simulink model "xPC_parker"  (Simulink 8.5)
settings: Solver=FixedStepDiscrete  StartTime=0.0  StopTime=inf  FixedStep=dts  RelTol=1e-3
InitFcn:
  | PARKER_DEPENDENCY
  | Parker_Multi_Axis_Init
  | Parker_ATI_Init
  | Parker_Home_Init
  | Parker_Davinci_Init
  | Parker_UDP_Init
  | Parker_LinIntPathPlan_Init
  | Parker_ScopeFormat_Init
  | Parker_magnetic_init
undefined symbols (not defined in the file): A, accel_filter_coeffs, ATI_torque_Nmm, B, counter_offset, DavinciFilterDen, DavinciFilterNum, DesiredPath, dt, dt_ENC, dt_trakstar, dts, dtudp, ENC_obs_filter_coeffs, encoder_counts, F, f_mag_desired_shape, filter_coeffs_bias, force_bias, forceDeadZone, FT_unbias_time, grav_vector, Home_in_TKbase, HOMING_dx, HOMING_num_joint, HOMING_tspan, HOMING_Vmov, inv_T, JOINT_Limits_Negative, JOINT_Limits_Postive, Kd, Ki_force, Kp, Kp_force, Kv_force, Low, N_acceleration, N_bias, N_ENC_obs_filter, N_obs_velocity, N_trakstar, N_velocity, Omega7IsLeftHanded, omni_scaling, PathPlanSpeed, pitch, quadrature_mode, R_FT2robot, R_omni, R_robot2TKbase, ResRateEpsilon, ResRateVelLimits, ResRateVelRatios, SafetyMargin, screw_pitch, torque_constant, trakstar_filter_coeffs, UDP_EN_Data2CMU, UDP_EN_DynAna, UDP_EN_VFRec ... (+6)
libraries: slrtlib x25, simulink x24, dspswit3 x15, xpcobsoletelib x15, xpcrtudplib x14, powerlib_meascontrol x3, xpcmeasurementcomputinglib x3, xpcconteclib x3
(part 1 of 3)
settings Model: Creator=Roger  LastModifiedBy=arma  CovSFcnEnable=off
settings SolverCC: EnableConcurrentExecution=on
settings OptimizationCC: BlockReduction=off  OptimizeBlockIOStorage=off  BufferReuse=off  GlobalBufferReuse=off  ExpressionFolding=off  LocalBlockOutputs=off  InitFltsAndDblsToZero=on
settings DebuggingCC: SolverPrmCheckMsg=warning  MultiTaskCondExecSysMsg=warning  MultiTaskRateTransMsg=warning  FcnCallInpInsideContextMsg=EnableAllAsWarning
settings HardwareCC: ProdIntDivRoundTo=Zero  ProdEndianess=LittleEndian  ProdLongLongMode=on  ProdHWDeviceType=Generic->32-bit x86 compatible
settings SFSimCC: SimParseCustomCode=off
settings RTWCC: SystemTargetFile=slrt.tlc  TemplateMakefile=slrt_default_tmf  Description=Simulink Real-Time  RTWCompilerOptimization=on
settings SimulinkRealTimeCC: GeneratePreprocessorConditionals=Disable all  xPCisDownloadable=off  xPCisModelTimeout=off  xPCModelTimeoutSecs=15

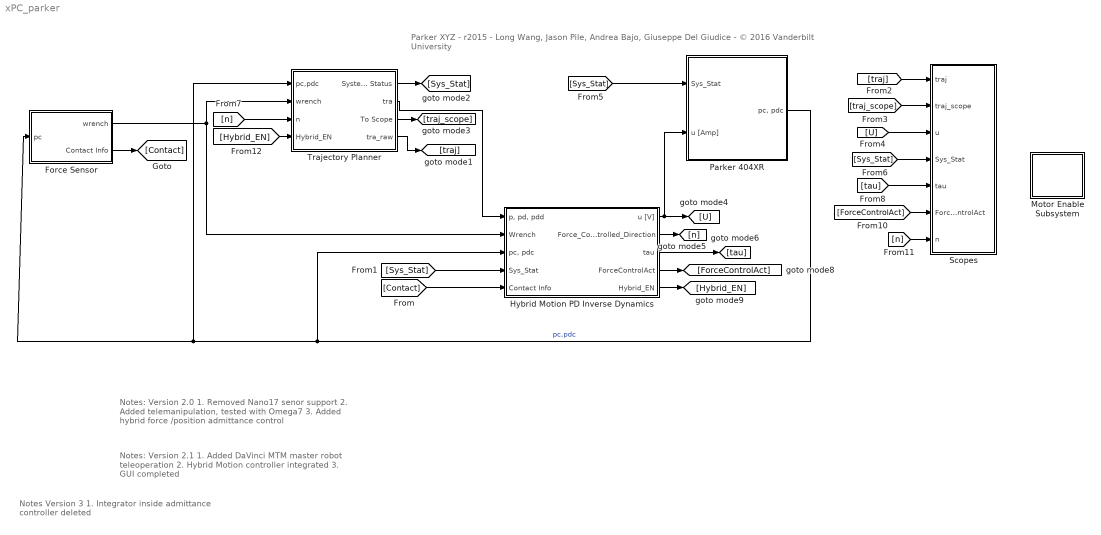
== system xPC_parker ==
  note: Notes Version 3
      | 1. Integrator inside admittance controller deleted
  note: Notes: Version 2.0
      | 1. Removed Nano17 senor support
      | 2. Added telemanipulation, tested with Omega7
      | 3. Added hybrid force /position admittance control
  note: Parker XYZ - r2015 - Long Wang, Jason Pile, Andrea Bajo, Giuseppe Del Giudice - © 2016 Vanderbilt University
  note: Notes: Version 2.1
      | 1. Added DaVinci MTM master robot teleoperation
      | 2. Hybrid Motion controller integrated
      | 3. GUI completed
  Force Sensor : Subsystem
  Hybrid Motion PD Inverse Dynamics : Subsystem  TreatAsAtomicUnit=on
  Motor Enable Subsystem : Subsystem
  Parker 404XR : Subsystem
  Scopes : Subsystem
  Trajectory Planner : Subsystem  TreatAsAtomicUnit=on
  wires:
  Hybrid Motion PD Inverse Dynamics/1(u [V]) -> [U], Parker 404XR/2(u [Amp])
  Parker 404XR/1("pc, pdc") -> Hybrid Motion PD Inverse Dynamics/3("pc, pdc"), Force Sensor/1(pc), Trajectory Planner/1(pc,pdc)  "pc,pdc"
  Trajectory Planner/2(tra) -> Hybrid Motion PD Inverse Dynamics/1("p, pd, pdd")
  Force Sensor/1(wrench) -> Hybrid Motion PD Inverse Dynamics/2(Wrench), Trajectory Planner/2(wrench)
  Trajectory Planner/1(System Status) -> [Sys_Stat]
  [Sys_Stat] -> Parker 404XR/1(Sys_Stat)
  [Sys_Stat] -> Hybrid Motion PD Inverse Dynamics/4(Sys_Stat)
  [traj] -> Scopes/1(traj)
  Trajectory Planner/3(To Scope) -> [traj_scope]
  [traj_scope] -> Scopes/2(traj_scope)
  [U] -> Scopes/3(u)
  [Sys_Stat] -> Scopes/4(Sys_Stat)
  Hybrid Motion PD Inverse Dynamics/2(Force_Controlled_Direction) -> [n]
  [n] -> Trajectory Planner/3(n)
  Hybrid Motion PD Inverse Dynamics/3(tau) -> [tau]
  [tau] -> Scopes/5(tau)
  Hybrid Motion PD Inverse Dynamics/4(ForceControlAct) -> [ForceControlAct]
  [ForceControlAct] -> Scopes/6(ForceControlAct)
  [n] -> Scopes/7(n)
  Hybrid Motion PD Inverse Dynamics/5(Hybrid_EN) -> [Hybrid_EN]
  [Hybrid_EN] -> Trajectory Planner/4(Hybrid_EN)
  Force Sensor/2(Contact Info) -> [Contact]
  [Contact] -> Hybrid Motion PD Inverse Dynamics/5(Contact Info)
  Trajectory Planner/4(tra_raw) -> [traj]

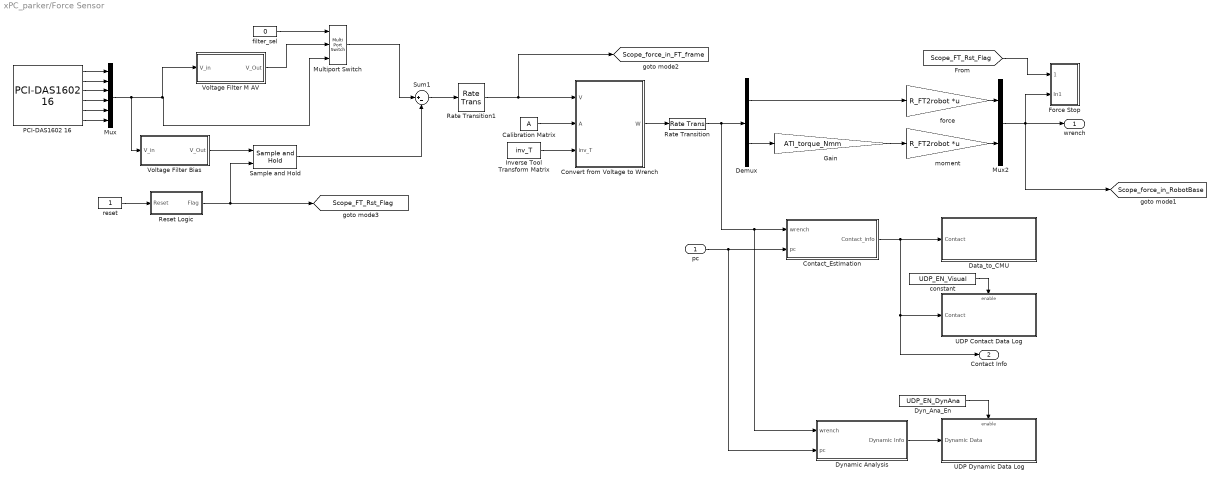
== system xPC_parker/Force Sensor ==
  pc : Inport
  Calibration Matrix : Constant  Value=A
  Contact_Estimation : Subsystem
  Convert from Voltage to Wrench : MATLAB Function  TreatAsAtomicUnit=on
  Data_to_CMU : Subsystem
  Demux : Demux  Outputs=2
  Dyn_Ana_En : Constant  Value=UDP_EN_DynAna
  Dynamic Analysis : Subsystem
  Force Stop : Subsystem
  Gain : Gain  Gain=ATI_torque_Nmm
  Inverse Tool Transform Matrix : Constant  Value=inv_T  VectorParams1D=off
  Multiport Switch : MultiPortSwitch  Inputs=2
  Mux : Mux  Inputs=6
  Mux2 : Mux  Inputs=2
  "PCI-DAS1602 16 " : xpcobsoletelib/Measurement Computing obs/A//D/PCI-DAS1602 16   channel=6  range=+-10V  mux=Differential (8 channels)  sampletime=dts  slot=-1
  Rate Transition : RateTransition  OutPortSampleTime=dt
  Rate Transition1 : RateTransition  OutPortSampleTime=dt
  Reset Logic : Subsystem
  Sample and Hold : powerlib_meascontrol/Additional Components/Sample and Hold  ic=zeros(6,1)  Ts=dts
  Sum1 : Sum  Inputs=|+-  SampleTime=dts
  UDP Contact Data Log : Subsystem
  UDP Dynamic Data Log : Subsystem
  Voltage Filter Bias : Subsystem
  Voltage Filter M AV : Subsystem
  constant : Constant  Value=UDP_EN_Visual
  filter_sel : Constant  Value=0
  force : Gain  Gain=R_FT2robot  Multiplication=Matrix(K*u)
  moment : Gain  Gain=R_FT2robot  Multiplication=Matrix(K*u)
  reset : Constant
  wrench : Outport
  Contact Info : Outport  Port=2
  tag scope: Scope_FT_Rst_Flag=global, Scope_force_in_FT_frame=global, Scope_force_in_RobotBase=global
  wires:
  "PCI-DAS1602 16 "/1 -> Mux/1
  "PCI-DAS1602 16 "/2 -> Mux/2
  "PCI-DAS1602 16 "/3 -> Mux/3
  "PCI-DAS1602 16 "/4 -> Mux/4
  "PCI-DAS1602 16 "/5 -> Mux/5
  Mux/1 -> Voltage Filter Bias/1(V_in), Voltage Filter M AV/1(V_in), Multiport Switch/3
  "PCI-DAS1602 16 "/6 -> Mux/6
  Calibration Matrix/1 -> Convert from Voltage to Wrench/2(A)
  Inverse Tool Transform Matrix/1 -> Convert from Voltage to Wrench/3(inv_T)
  Sum1/1 -> Rate Transition1/1
  Demux/1 -> force/1
  Demux/2 -> Gain/1
  force/1 -> Mux2/1
  moment/1 -> Mux2/2
  Mux2/1 -> [Scope_force_in_RobotBase], wrench/1, Force Stop/2(In1)
  Convert from Voltage to Wrench/1(W) -> Rate Transition/1
  Rate Transition/1 -> Dynamic Analysis/1(wrench), Contact_Estimation/1(wrench), Demux/1
  Multiport Switch/1 -> Sum1/1
  filter_sel/1 -> Multiport Switch/1
  Contact_Estimation/1(Contact_info) -> Contact Info/1, UDP Contact Data Log/1(Contact), Data_to_CMU/1(Contact)
  pc/1 -> Dynamic Analysis/2(pc), Contact_Estimation/2(pc)
  Voltage Filter Bias/1(V_Out) -> Sample and Hold/1
  Sample and Hold/1 -> Sum1/2
  reset/1 -> Reset Logic/1(Reset)
  Reset Logic/1(Flag) -> [Scope_FT_Rst_Flag], Sample and Hold/2
  Dynamic Analysis/1(Dynamic Info) -> UDP Dynamic Data Log/1(Dynamic Data)
  Dyn_Ana_En/1 -> UDP Dynamic Data Log/Enable
  Rate Transition1/1 -> [Scope_force_in_FT_frame], Convert from Voltage to Wrench/1(V)
  Voltage Filter M AV/1(V_Out) -> Multiport Switch/2
  constant/1 -> UDP Contact Data Log/Enable
  [Scope_FT_Rst_Flag] -> Force Stop/1(ResetFlag)
  Gain/1 -> moment/1

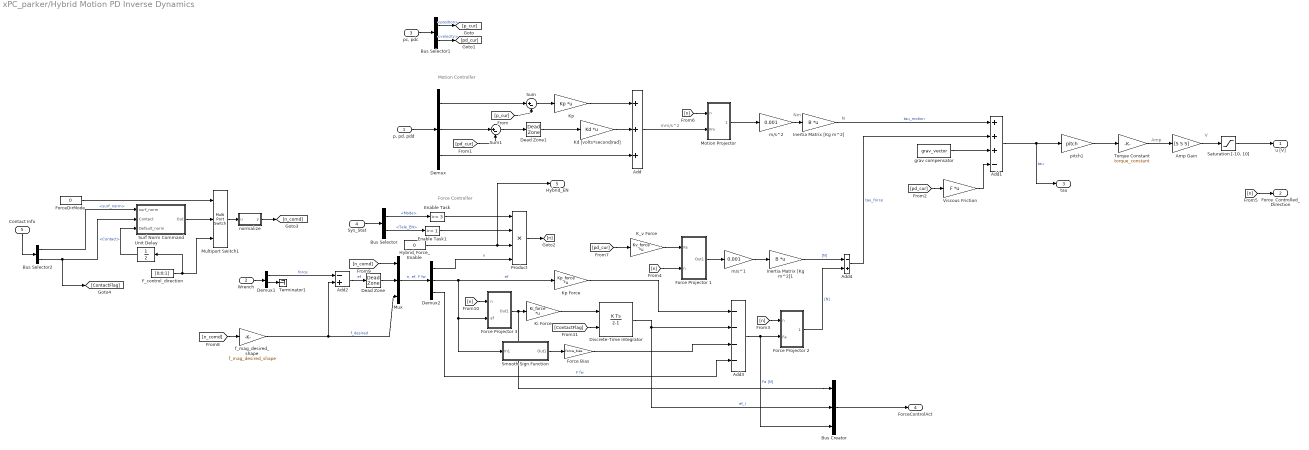
== system xPC_parker/Hybrid Motion PD Inverse Dynamics ==
  note: Force Controller
  note: Motion Controller
  note: N
  note: mm/s^2
  note: Amp
  note: V
  note: Nm
  "p, pd, pdd" : Inport
  Wrench : Inport  Port=2
  "pc, pdc" : Inport  Port=3
  Sys_Stat : Inport  Port=4
  Contact Info : Inport  Port=5
  Add : Sum  Inputs=+++
  Add1 : Sum  Inputs=+++-  SampleTime=dt
  Add2 : Sum  Inputs=-+
  Add3 : Sum  Inputs=----
  Add4 : Sum  Inputs=-+
  Amp Gain : Gain  Gain=[5 5 5]
  Bus Creator : BusCreator  Inputs=3
  Bus Selector : BusSelector  OutputSignals=Mode,Tele_EN
  Bus Selector1 : BusSelector  OutputSignals=position,velocity
  Bus Selector2 : BusSelector  OutputSignals=surf_norm,Contact
  Dead Zone : DeadZone  LowerValue=-0.02  UpperValue=0.02  SaturateOnIntegerOverflow=on
  Dead Zone1 : DeadZone  LowerValue=-2.5  UpperValue=2.5  SaturateOnIntegerOverflow=on
  Demux : Demux  Outputs=[3 3 3]
  Demux1 : Demux  Outputs=2
  Demux2 : Demux  Outputs=3
  Discrete-Time Integrator : DiscreteIntegrator  ExternalReset=falling  SampleTime=dt  UpperSaturationLimit=20  LowerSaturationLimit=-20
  Enable Task : simulink/Logic and Bit Operations/Compare To Constant  relop=>=  const=3  OutDataTypeStr=boolean
  Enable Task1 : simulink/Logic and Bit Operations/Compare To Constant  relop=>=  const=1  OutDataTypeStr=boolean
  F_control_direction : Constant  Value=[0;0;1]
  Force Bias : Gain  Gain=force_bias  SampleTime=dt
  Force Projector 1 : Subsystem  TreatAsAtomicUnit=on
  Force Projector 2 : Subsystem  TreatAsAtomicUnit=on
  Force Projector 3 : Subsystem  TreatAsAtomicUnit=on
  ForceDirMode : Constant  Value=0
  Hybrid_Force_Enable : Constant  Value=0
  Inertia Matrix [Kg m^2] : Gain  Gain=B  Multiplication=Matrix(K*u)
  Inertia Matrix [Kg m^2]1 : Gain  Gain=B  Multiplication=Matrix(K*u)
  K_v Force : Gain  Gain=Kv_force  Multiplication=Matrix(K*u)  SampleTime=dt
  Kd [volts*second/rad] : Gain  Gain=Kd  Multiplication=Matrix(K*u)
  Ki Force : Gain  Gain=Ki_force  Multiplication=Matrix(K*u)  SampleTime=dt
  Kp : Gain  Gain=Kp  Multiplication=Matrix(K*u)
  Kp Force : Gain  Gain=Kp_force  Multiplication=Matrix(K*u)  SampleTime=dt
  Motion Projector : Subsystem  TreatAsAtomicUnit=on
  Multiport Switch1 : MultiPortSwitch  Inputs=2
  Mux : Mux  Inputs=3
  Product : Product  Inputs=4  RndMeth=Zero
  "Saturation [-10, 10]" : Saturate  UpperLimit=10  LowerLimit=-10
  Smooth Sign Function : Subsystem
  Sum : Sum  Inputs=|+-
  Sum1 : Sum  Inputs=|+-
  Surf Norm Command : Subsystem
  Terminator1 : Terminator
  Torque Constant : Gain  Gain=torque_constant
  Unit Delay : UnitDelay  InitialCondition=[0;0;1]  SampleTime=-1
  Viscous Friction : Gain  Gain=F  Multiplication=Matrix(K*u)  SampleTime=dt
  f_mag_desired_shape : Gain  Gain=f_mag_desired_shape
  grav compensator : Constant  Value=grav_vector
  m/s^1 : Gain  Gain=0.001
  m/s^2 : Gain  Gain=0.001
  normalize : MATLAB Function  TreatAsAtomicUnit=on
  pitch1 : Gain  Gain=pitch
  u [V] : Outport
  Force_Controlled_Direction : Outport  Port=2
  tau : Outport  Port=3
  ForceControlAct : Outport  Port=4
  Hybrid_EN : Outport  Port=5
  wires:
  "Saturation [-10, 10]"/1 -> u [V]/1
  m/s^2/1 -> Inertia Matrix [Kg m^2]/1
  Torque Constant/1 -> Amp Gain/1
  Add1/1 -> tau/1, pitch1/1  "tau"
  pitch1/1 -> Torque Constant/1
  Amp Gain/1 -> "Saturation [-10, 10]"/1
  "p, pd, pdd"/1 -> Demux/1
  "pc, pdc"/1 -> Bus Selector1/1
  Sum/1 -> Kp/1
  Demux/1 -> Sum/1
  Demux/2 -> Sum1/1
  Bus Selector1/1 -> [p_cur]  "<position>"
  [p_cur] -> Sum/2
  [pd_cur] -> Sum1/2
  [pd_cur] -> Viscous Friction/1
  Bus Selector1/2 -> [pd_cur]  "<velocity>"
  Kp/1 -> Add/1
  Kd [volts*second/rad]/1 -> Add/2
  Demux/3 -> Add/3
  Add/1 -> Motion Projector/2(Fm)
  Motion Projector/1(Out1) -> m/s^2/1
  Ki Force/1 -> Discrete-Time Integrator/1
  Discrete-Time Integrator/1 -> Bus Creator/2, Add3/2  "ef_I"
  Demux2/2 -> Kp Force/1, Force Projector 3/2(ef), Smooth Sign Function/1(In1)  "ef"
  Kp Force/1 -> Add3/1
  Add3/1 -> Bus Creator/3, Force Projector 2/2(Fa)  "Fa [N]"
  Force Projector 1/1(Out1) -> m/s^1/1
  K_v Force/1 -> Force Projector 1/1(Fa)
  m/s^1/1 -> Inertia Matrix [Kg m^2]1/1
  Inertia Matrix [Kg m^2]1/1 -> Add4/1  "[N]"
  Force Projector 2/1(Out1) -> Add4/2  "[N]"
  Smooth Sign Function/1(Out1) -> Force Bias/1
  Force Bias/1 -> Add3/3
  Demux2/3 -> Add3/4  "F fw"
  [n] -> Force Projector 2/1(n)
  [n] -> Force Projector 1/2(n)
  [pd_cur] -> K_v Force/1
  Inertia Matrix [Kg m^2]/1 -> Add1/1  "tau_motion"
  Add4/1 -> Add1/2  "tau_force"
  grav compensator/1 -> Add1/3
  Viscous Friction/1 -> Add1/4
  f_mag_desired_shape/1 -> Add2/2, Mux/3  "f_desired"
  Add2/1 -> Dead Zone/1  "ef"
  Mux/1 -> Demux2/1  "n, ef, F fw"
  [n] -> Motion Projector/1(n)
  Wrench/1 -> Demux1/1
  Demux1/2 -> Terminator1/1
  Demux1/1 -> Add2/1  "force"
  Sys_Stat/1 -> Bus Selector/1
  Bus Selector/1 -> Enable Task/1  "<Mode>"
  Enable Task/1 -> Product/1
  Bus Selector/2 -> Enable Task1/1  "<Tele_EN>"
  [n] -> Force_Controlled_Direction/1
  Product/1 -> [n]
  Enable Task1/1 -> Product/2
  Demux2/1 -> Product/4  "n"
  Dead Zone/1 -> Mux/2
  Contact Info/1 -> Bus Selector2/1
  F_control_direction/1 -> Unit Delay/1, Multiport Switch1/3
  ForceDirMode/1 -> Multiport Switch1/1
  Multiport Switch1/1 -> normalize/1(u)
  normalize/1(y) -> [n_comd]
  [n_comd] -> f_mag_desired_shape/1
  [n_comd] -> Mux/1
  Force Projector 3/1(Out1) -> Bus Creator/1, Ki Force/1
  [n] -> Force Projector 3/1(n)
  Sum1/1 -> Dead Zone1/1
  Dead Zone1/1 -> Kd [volts*second/rad]/1
  Bus Creator/1 -> ForceControlAct/1
  Bus Selector2/2 -> Surf Norm Command/2(Contact), [ContactFlag]  "<Contact>"
  [ContactFlag] -> Discrete-Time Integrator/2
  Bus Selector2/1 -> Surf Norm Command/1(surf_norm)  "<surf_norm>"
  Surf Norm Command/1(Out) -> Multiport Switch1/2
  Unit Delay/1 -> Surf Norm Command/3(Default_norm)
  Hybrid_Force_Enable/1 -> Product/3, Hybrid_EN/1

== system xPC_parker/Motor Enable Subsystem ==
  Demux : Demux  Outputs=3
  Enable Motors : Constant  Value=ones(3,1)
  PCI-DDA08 12  to PORTA : xpcmeasurementcomputinglib/Digital Output/PCI-DDA08 12   channel=[4 5 6]  port=A  reset=[1 1 1]  initValue=[0 0 0]  chip=1  sampletime=dt  slot=-1
  wires:
  Demux/1 -> PCI-DDA08 12  to PORTA/1
  Demux/2 -> PCI-DDA08 12  to PORTA/2
  Demux/3 -> PCI-DDA08 12  to PORTA/3
  Enable Motors/1 -> Demux/1

== system xPC_parker/Parker 404XR ==
  Sys_Stat : Inport
  u [Amp] : Inport  Port=2
  Bus Creator : BusCreator  Inputs=5
  Bus Selector : BusSelector  OutputSignals=Enc_Reset
  Count to Position : Subsystem
  Magnetic Tracker 125 Hz : Subsystem  TreatAsAtomicUnit=on
      mask Display: %image(imread('trakSTAR.jpg'));
  Plant : Subsystem
  "pc, pdc" : Outport
  tag scope: Scope_p_cur=global
  wires:
  Count to Position/1(position) -> Bus Creator/1  "position"
  Plant/1(counts) -> Count to Position/1(count)
  u [Amp]/1 -> Plant/1(u)
  Bus Creator/1 -> [Scope_p_cur], "pc, pdc"/1
  Count to Position/2(velocity) -> Bus Creator/2  "velocity"
  Plant/2(LimitSW) -> Bus Creator/4  "LimitSW"
  Sys_Stat/1 -> Bus Selector/1
  Bus Selector/1 -> Count to Position/2(EncoderReset)  "<Enc_Reset>"
  Count to Position/3(acceleration) -> Bus Creator/3  "acceleration"
  Magnetic Tracker 125 Hz/1(TrakStar) -> Bus Creator/5

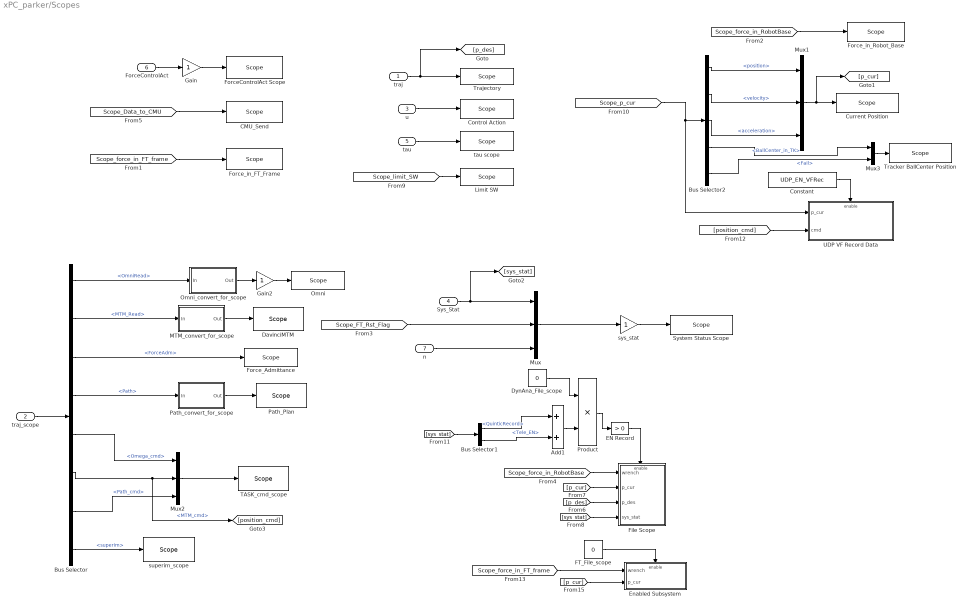
== system xPC_parker/Scopes ==
  traj : Inport
  traj_scope : Inport  Port=2
  u : Inport  Port=3
  Sys_Stat : Inport  Port=4
  tau : Inport  Port=5
  ForceControlAct : Inport  Port=6
  n : Inport  Port=7
  Add1 : Sum  SampleTime=dt
  Bus Selector : BusSelector  OutputSignals=OmniRead,MTM_Read,ForceAdm,Path,Omega_cmd,MTM_cmd,Path_cmd,superim
  Bus Selector1 : BusSelector  OutputSignals=QuinticRecord,Tele_EN
  Bus Selector2 : BusSelector  OutputSignals=position,velocity,acceleration,Tracker.BallCenter_in_TK,Tracker.Fail
  CMU_Send : slrtlib/Displays and Logging/Scope   scopeno=5  scopetype=Host  autostart=on  viewmode=Numerical  formatstr=CMU_force_scope  grid=on  ylimits=[0,0]  nosamples=Scope_Samples  noprepostsamples=0  interleave=1  triggermode=FreeRun  triggersignal=1  trigsignalfromport=off  triggerlevel=0.0  triggerslope=Either  triggerscope=1  triggersample=0  filename=data.dat  mode=Lazy  writesize=512  autorestart=off  dynamicfilemode=off  maxwritefilesize=512*1024^2
  Constant : Constant  Value=UDP_EN_VFRec
  Control Action : slrtlib/Displays and Logging/Scope   scopeno=2  scopetype=Target  autostart=on  viewmode=Numerical  formatstr=Control_Vals_format  grid=on  ylimits=[0,0]  nosamples=Scope_Samples  noprepostsamples=0  interleave=5  triggermode=FreeRun  triggersignal=1  trigsignalfromport=off  triggerlevel=0.0  triggerslope=Either  triggerscope=1  triggersample=0  filename=data.dat  mode=Lazy  writesize=512  autorestart=off  dynamicfilemode=off  maxwritefilesize=512*1024^2
  Current Position : slrtlib/Displays and Logging/Scope   scopeno=10  scopetype=Target  autostart=on  viewmode=Numerical  formatstr=Current_Position_Vals_format  grid=on  ylimits=[0,0]  nosamples=Scope_Samples  noprepostsamples=0  interleave=1  triggermode=FreeRun  triggersignal=1  trigsignalfromport=off  triggerlevel=0.0  triggerslope=Either  triggerscope=1  triggersample=0  filename=data.dat  mode=Lazy  writesize=512  autorestart=off  dynamicfilemode=off  maxwritefilesize=512*1024^2
  DavinciMTM : slrtlib/Displays and Logging/Scope   scopeno=4  scopetype=Host  autostart=on  viewmode=Numerical  formatstr=MTM_udp_scope_format  grid=on  ylimits=[0,0]  nosamples=50  noprepostsamples=0  interleave=1  triggermode=FreeRun  triggersignal=1  trigsignalfromport=off  triggerlevel=0.0  triggerslope=Either  triggerscope=1  triggersample=0  filename=data.dat  mode=Lazy  writesize=512  autorestart=off  dynamicfilemode=off  maxwritefilesize=512*1024^2
  DynAna_File_scope : Constant  Value=0
  EN Record : simulink/Logic and Bit Operations/Compare To Constant  relop=>  const=0  OutDataTypeStr=boolean
  Enabled Subsystem : Subsystem  TreatAsAtomicUnit=on
  FT_File_scope : Constant  Value=0
  File Scope : Subsystem
  ForceControlAct Scope : slrtlib/Displays and Logging/Scope   scopeno=18  scopetype=Host  autostart=on  viewmode=Numerical  formatstr=ForceControlAct_Scope  grid=on  ylimits=[0,0]  nosamples=Scope_Samples  noprepostsamples=0  interleave=1  triggermode=FreeRun  triggersignal=1  trigsignalfromport=off  triggerlevel=0.0  triggerslope=Either  triggerscope=1  triggersample=0  filename=data.dat  mode=Lazy  writesize=512  autorestart=off  dynamicfilemode=off  maxwritefilesize=512*1024^2
  Force_Admittance : slrtlib/Displays and Logging/Scope   scopeno=8  scopetype=Host  autostart=on  viewmode=Numerical  formatstr=forceAdmitFormat  grid=on  ylimits=[0,0]  nosamples=250  noprepostsamples=0  interleave=1  triggermode=FreeRun  triggersignal=1  trigsignalfromport=off  triggerlevel=0.0  triggerslope=Either  triggerscope=1  triggersample=0  filename=data.dat  mode=Lazy  writesize=512  autorestart=off  dynamicfilemode=off  maxwritefilesize=512*1024^2
  Force_in_FT_Frame : slrtlib/Displays and Logging/Scope   scopeno=6  scopetype=Host  autostart=on  viewmode=Numerical  formatstr=forceFormat  grid=on  ylimits=[0,0]  nosamples=Scope_Samples  noprepostsamples=0  interleave=1  triggermode=FreeRun  triggersignal=1  trigsignalfromport=off  triggerlevel=0.0  triggerslope=Either  triggerscope=1  triggersample=0  filename=data.dat  mode=Lazy  writesize=512  autorestart=off  dynamicfilemode=off  maxwritefilesize=512*1024^2
  Force_in_Robot_Base : slrtlib/Displays and Logging/Scope   scopeno=7  scopetype=Target  autostart=on  viewmode=Numerical  formatstr=forceFormat  grid=on  ylimits=[0,0]  nosamples=Scope_Samples  noprepostsamples=0  interleave=1  triggermode=FreeRun  triggersignal=1  trigsignalfromport=off  triggerlevel=0.0  triggerslope=Either  triggerscope=1  triggersample=0  filename=data.dat  mode=Lazy  writesize=512  autorestart=off  dynamicfilemode=off  maxwritefilesize=512*1024^2
  Gain : Gain
  Gain2 : Gain
  Limit SW : slrtlib/Displays and Logging/Scope   scopeno=9  scopetype=Host  autostart=on  viewmode=Numerical  formatstr=limitSwitchFormat  grid=on  ylimits=[0,0]  nosamples=250  noprepostsamples=0  interleave=1  triggermode=FreeRun  triggersignal=1  trigsignalfromport=off  triggerlevel=0.0  triggerslope=Either  triggerscope=1  triggersample=0  filename=data.dat  mode=Lazy  writesize=512  autorestart=off  dynamicfilemode=off  maxwritefilesize=512*1024^2
  MTM_convert_for_scope : Subsystem
  Mux : Mux  Inputs=3
  Mux1 : Mux  Inputs=3
  Mux2 : Mux  Inputs=3
  Mux3 : Mux  Inputs=2
  Omni : slrtlib/Displays and Logging/Scope   scopeno=3  scopetype=Host  autostart=on  viewmode=Numerical  formatstr=omniFormat  grid=on  ylimits=[0,0]  nosamples=50  noprepostsamples=0  interleave=1  triggermode=FreeRun  triggersignal=1  trigsignalfromport=off  triggerlevel=0.0  triggerslope=Either  triggerscope=1  triggersample=0  filename=data.dat  mode=Lazy  writesize=512  autorestart=off  dynamicfilemode=off  maxwritefilesize=512*1024^2
  Omni_convert_for_scope : Subsystem
  Path_Plan : slrtlib/Displays and Logging/Scope   scopeno=17  scopetype=Host  autostart=on  viewmode=Numerical  formatstr=Scope_format_Path  grid=on  ylimits=[0,0]  nosamples=50  noprepostsamples=0  interleave=1  triggermode=FreeRun  triggersignal=1  trigsignalfromport=off  triggerlevel=0.0  triggerslope=Either  triggerscope=1  triggersample=0  filename=data.dat  mode=Lazy  writesize=512  autorestart=off  dynamicfilemode=off  maxwritefilesize=512*1024^2
  Path_convert_for_scope : Subsystem
  Product : Product  RndMeth=Zero
  System Status Scope : slrtlib/Displays and Logging/Scope   scopeno=11  scopetype=Target  autostart=on  viewmode=Numerical  formatstr=Scope_format_sys_stat  grid=on  ylimits=[0,0]  nosamples=Scope_Samples  noprepostsamples=0  interleave=1  triggermode=FreeRun  triggersignal=1  trigsignalfromport=off  triggerlevel=0.0  triggerslope=Either  triggerscope=1  triggersample=0  filename=data.dat  mode=Lazy  writesize=512  autorestart=off  dynamicfilemode=off  maxwritefilesize=512*1024^2
  TASK_cmd_scope : slrtlib/Displays and Logging/Scope   scopeno=15  scopetype=Host  autostart=on  viewmode=Numerical  formatstr=Scope_format_TASK_cmd  grid=on  ylimits=[0,0]  nosamples=50  noprepostsamples=0  interleave=1  triggermode=FreeRun  triggersignal=1  trigsignalfromport=off  triggerlevel=0.0  triggerslope=Either  triggerscope=1  triggersample=0  filename=data.dat  mode=Lazy  writesize=512  autorestart=off  dynamicfilemode=off  maxwritefilesize=512*1024^2
  Tracker BallCenter Position : slrtlib/Displays and Logging/Scope   scopeno=21  scopetype=Host  autostart=on  viewmode=Numerical  formatstr=Scope_format_Tracker_BallCenter  grid=on  ylimits=[0,0]  nosamples=Scope_Samples  noprepostsamples=0  interleave=1  triggermode=FreeRun  triggersignal=1  trigsignalfromport=off  triggerlevel=0.0  triggerslope=Either  triggerscope=1  triggersample=0  filename=data.dat  mode=Lazy  writesize=512  autorestart=off  dynamicfilemode=off  maxwritefilesize=512*1024^2
  Trajectory : slrtlib/Displays and Logging/Scope   scopeno=1  scopetype=Target  autostart=on  viewmode=Numerical  formatstr=p_cmd_scope_format  grid=on  ylimits=[0,0]  nosamples=25  noprepostsamples=0  interleave=1  triggermode=FreeRun  triggersignal=1  trigsignalfromport=off  triggerlevel=0.0  triggerslope=Either  triggerscope=1  triggersample=0  filename=foamdata1.dat  mode=Lazy  writesize=512  autorestart=off  dynamicfilemode=off  maxwritefilesize=512*1024^2
  UDP VF Record Data : Subsystem
  superim_scope : slrtlib/Displays and Logging/Scope   scopeno=19  scopetype=Host  autostart=on  viewmode=Numerical  formatstr=Scope_format_superim  grid=on  ylimits=[0,0]  nosamples=50  noprepostsamples=0  interleave=1  triggermode=FreeRun  triggersignal=1  trigsignalfromport=off  triggerlevel=0.0  triggerslope=Either  triggerscope=1  triggersample=0  filename=data.dat  mode=Lazy  writesize=512  autorestart=off  dynamicfilemode=off  maxwritefilesize=512*1024^2
  sys_stat : Gain
  tau scope : slrtlib/Displays and Logging/Scope   scopeno=12  scopetype=Host  autostart=on  viewmode=Numerical  formatstr=Scope_format_tau  grid=on  ylimits=[0,0]  nosamples=Scope_Samples  noprepostsamples=0  interleave=1  triggermode=FreeRun  triggersignal=1  trigsignalfromport=off  triggerlevel=0.0  triggerslope=Either  triggerscope=1  triggersample=0  filename=data.dat  mode=Lazy  writesize=512  autorestart=off  dynamicfilemode=off  maxwritefilesize=512*1024^2
  wires:
  [Scope_Data_to_CMU] -> CMU_Send/1
  [Scope_force_in_FT_frame] -> Force_in_FT_Frame/1
  [Scope_force_in_RobotBase] -> Force_in_Robot_Base/1
  traj/1 -> [p_des], Trajectory/1
  Bus Selector/1 -> Omni_convert_for_scope/1(In)  "<OmniRead>"
  Bus Selector/3 -> Force_Admittance/1  "<ForceAdm>"
  u/1 -> Control Action/1
  [Scope_limit_SW] -> Limit SW/1
  traj_scope/1 -> Bus Selector/1
  Bus Selector/2 -> MTM_convert_for_scope/1(In)  "<MTM_Read>"
  MTM_convert_for_scope/1(Out) -> DavinciMTM/1
  Omni_convert_for_scope/1(Out) -> Gain2/1
  Sys_Stat/1 -> Mux/1, [sys_stat]
  Gain2/1 -> Omni/1
  tau/1 -> tau scope/1
  [Scope_FT_Rst_Flag] -> Mux/2
  Mux/1 -> sys_stat/1
  Mux1/1 -> [p_cur], Current Position/1
  Bus Selector/4 -> Path_convert_for_scope/1(In)  "<Path>"
  Path_convert_for_scope/1(Out) -> Path_Plan/1
  [Scope_force_in_RobotBase] -> File Scope/1(wrench)
  [p_cur] -> File Scope/2(p_cur)
  [p_des] -> File Scope/3(p_des)
  [sys_stat] -> File Scope/4(sys_stat)
  [sys_stat] -> Bus Selector1/1
  Bus Selector1/2 -> Add1/2  "<Tele_EN>"
  EN Record/1 -> File Scope/Enable
  [Scope_p_cur] -> UDP VF Record Data/1(p_cur), Bus Selector2/1
  Bus Selector2/1 -> Mux1/1  "<position>"
  Bus Selector2/2 -> Mux1/2  "<velocity>"
  Bus Selector2/3 -> Mux1/3  "<acceleration>"
  Bus Selector1/1 -> Add1/1  "<QuinticRecord>"
  DynAna_File_scope/1 -> Product/1
  Add1/1 -> Product/2
  Product/1 -> EN Record/1
  ForceControlAct/1 -> Gain/1
  Gain/1 -> ForceControlAct Scope/1
  Bus Selector/6 -> [position_cmd], Mux2/2  "<MTM_cmd>"
  Bus Selector/7 -> Mux2/3  "<Path_cmd>"
  Bus Selector/5 -> Mux2/1  "<Omega_cmd>"
  Mux2/1 -> TASK_cmd_scope/1
  [position_cmd] -> UDP VF Record Data/2(cmd)
  Constant/1 -> UDP VF Record Data/Enable
  Bus Selector/8 -> superim_scope/1  "<superim>"
  sys_stat/1 -> System Status Scope/1
  Bus Selector2/5 -> Mux3/2  "<Fail>"
  Bus Selector2/4 -> Mux3/1  "<BallCenter_in_TK>"
  Mux3/1 -> Tracker BallCenter Position/1
  n/1 -> Mux/3
  [Scope_force_in_FT_frame] -> Enabled Subsystem/1(wrench)
  [p_cur] -> Enabled Subsystem/2(p_cur)
  FT_File_scope/1 -> Enabled Subsystem/Enable

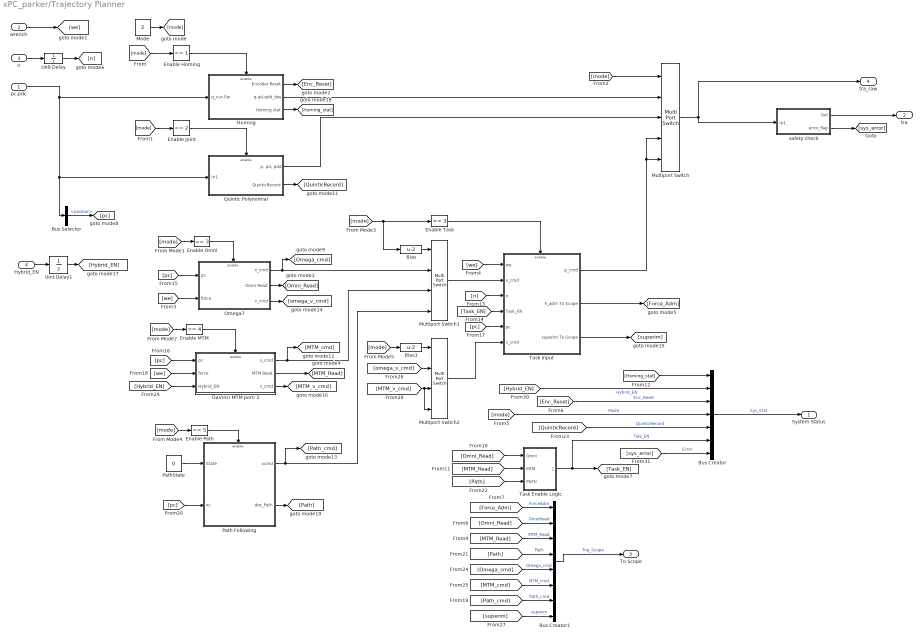
== system xPC_parker/Trajectory Planner ==
  pc,pdc : Inport
  wrench : Inport  Port=2
  n : Inport  Port=3
  Hybrid_EN : Inport  Port=4
  Bias : Bias  Bias=-2
  Bias1 : Bias  Bias=-2
  Bus Creator : BusCreator  Inputs=7
  Bus Creator1 : BusCreator  Inputs=8
  Bus Selector : BusSelector  OutputSignals=position
  DaVinci MTM port: 2 : Subsystem
  Enable Homing : simulink/Logic and Bit Operations/Compare To Constant  relop===  const=1  OutDataTypeStr=boolean
  Enable Joint : simulink/Logic and Bit Operations/Compare To Constant  relop===  const=2  OutDataTypeStr=boolean
  Enable MTM : simulink/Logic and Bit Operations/Compare To Constant  relop===  const=4  OutDataTypeStr=boolean
  Enable Omni : simulink/Logic and Bit Operations/Compare To Constant  relop===  const=3  OutDataTypeStr=boolean
  Enable Path : simulink/Logic and Bit Operations/Compare To Constant  relop===  const=5  OutDataTypeStr=boolean
  Enable Task : simulink/Logic and Bit Operations/Compare To Constant  relop=>=  const=3  OutDataTypeStr=boolean
  Homing : Subsystem
  Mode : Constant  Value=2
  Multiport Switch : MultiPortSwitch  Inputs=4
  Multiport Switch1 : MultiPortSwitch
  Multiport Switch2 : MultiPortSwitch
  Omega7 : Subsystem
  Path Following : Subsystem
  PathState : Constant  Value=0
  Quintic Polynomial : Subsystem  TreatAsAtomicUnit=on
  Task Enable Logic : Subsystem
  Task Input : Subsystem  TreatAsAtomicUnit=on
  Unit Delay : UnitDelay  InitialCondition=zeros(3,1)  SampleTime=-1
  Unit Delay1 : UnitDelay  SampleTime=-1
  safety check : Subsystem
  System Status : Outport
  tra : Outport  Port=2
  To Scope : Outport  Port=3
  tra_raw : Outport  Port=4
  wires:
  pc,pdc/1 -> Bus Selector/1, Quintic Polynomial/1(In1), Homing/1(q_cur,Sw)
  Enable Joint/1 -> Quintic Polynomial/Enable
  Homing/2(q,qd,qdd_des) -> Multiport Switch/2
  Quintic Polynomial/1("p, pd, pdd") -> Multiport Switch/3
  Enable Homing/1 -> Homing/Enable
  Mode/1 -> [mode]
  [mode] -> Enable Homing/1
  [mode] -> Enable Joint/1
  [mode] -> Multiport Switch/1
  Omega7/1(x_cmd) -> [Omega_cmd], Multiport Switch1/2
  Enable Task/1 -> Task Input/Enable
  Task Input/1(p_cmd) -> Multiport Switch/4, Multiport Switch/5
  Bus Selector/1 -> [pc]  "<position>"
  Multiport Switch1/1 -> Task Input/2(x_cmd)
  Bias/1 -> Multiport Switch1/1
  [mode] -> Enable Omni/1
  Enable Omni/1 -> Omega7/Enable
  [mode] -> Bias/1, Enable Task/1
  DaVinci MTM port: 2/1(x_cmd) -> [MTM_cmd], Multiport Switch1/3
  [mode] -> Enable MTM/1
  Enable MTM/1 -> DaVinci MTM port: 2/Enable
  wrench/1 -> [we]
  [we] -> Task Input/1(we)
  [we] -> Omega7/2(force)
  Bus Creator/1 -> System Status/1  "Sys_Stat"
  Homing/1(Encoder Reset) -> [Enc_Reset]
  [mode] -> Bus Creator/4  "Mode"
  [Enc_Reset] -> Bus Creator/3  "Enc_Reset"
  Bus Creator1/1 -> To Scope/1  "Traj_Scope"
  Omega7/2(Omni Read) -> [Omni_Read]
  DaVinci MTM port: 2/2(MTM Read) -> [MTM_Read]
  Task Input/2(F_adm To Scope) -> [Force_Adm]
  [Force_Adm] -> Bus Creator1/1  "ForceAdm"
  [Omni_Read] -> Bus Creator1/2  "OmniRead"
  [MTM_Read] -> Bus Creator1/3  "MTM_Read"
  [Omni_Read] -> Task Enable Logic/1(Omni)
  [MTM_Read] -> Task Enable Logic/2(MTM)
  Task Enable Logic/1(TeleEN) -> Bus Creator/6, [Task_EN]  "Tele_EN"
  [n] -> Task Input/3(n)
  n/1 -> Unit Delay/1
  Unit Delay/1 -> [n]
  [Task_EN] -> Task Input/4(Task_EN)
  [pc] -> Omega7/1(pc)
  [pc] -> DaVinci MTM port: 2/1(pc)
  [pc] -> Task Input/5(pc)
  [we] -> DaVinci MTM port: 2/2(force)
  PathState/1 -> Path Following/1(State)
  [pc] -> Path Following/2(xc)
  [mode] -> Enable Path/1
  Enable Path/1 -> Path Following/Enable
  Path Following/1(xcmd) -> Multiport Switch1/4, [Path_cmd]
  Path Following/2(des_Path) -> [Path]
  [Path] -> Bus Creator1/4  "Path"
  [Path] -> Task Enable Logic/3(PATH)
  Quintic Polynomial/2(QuinticRecord) -> [QuinticRecord]
  [QuinticRecord] -> Bus Creator/5  "QuinticRecord"
  [Omega_cmd] -> Bus Creator1/5  "Omega_cmd"
  [Path_cmd] -> Bus Creator1/7  "Path_cmd"
  [MTM_cmd] -> Bus Creator1/6  "MTM_cmd"
  Omega7/3(v_cmd) -> [omega_v_cmd]
  Task Input/3(superim To Scope) -> [superim]
  [superim] -> Bus Creator1/8  "superim"
  DaVinci MTM port: 2/3(v_cmd) -> [MTM_v_cmd]
  [omega_v_cmd] -> Multiport Switch2/2
  [MTM_v_cmd] -> Multiport Switch2/4, Multiport Switch2/3
  Bias1/1 -> Multiport Switch2/1
  [mode] -> Bias1/1
  Multiport Switch2/1 -> Task Input/6(v_cmd)
  Hybrid_EN/1 -> Unit Delay1/1
  [Hybrid_EN] -> DaVinci MTM port: 2/3(Hybrid_EN)
  [Hybrid_EN] -> Bus Creator/2  "Hybrid_EN"
  Unit Delay1/1 -> [Hybrid_EN]
  Homing/3(Homing stat) -> [Homing_stat]
  [Homing_stat] -> Bus Creator/1
  Multiport Switch/1 -> tra_raw/1, safety check/1(In1)
  safety check/1(Out) -> tra/1
  safety check/2(error_flag) -> [sys_error]
  [sys_error] -> Bus Creator/7  "Error"

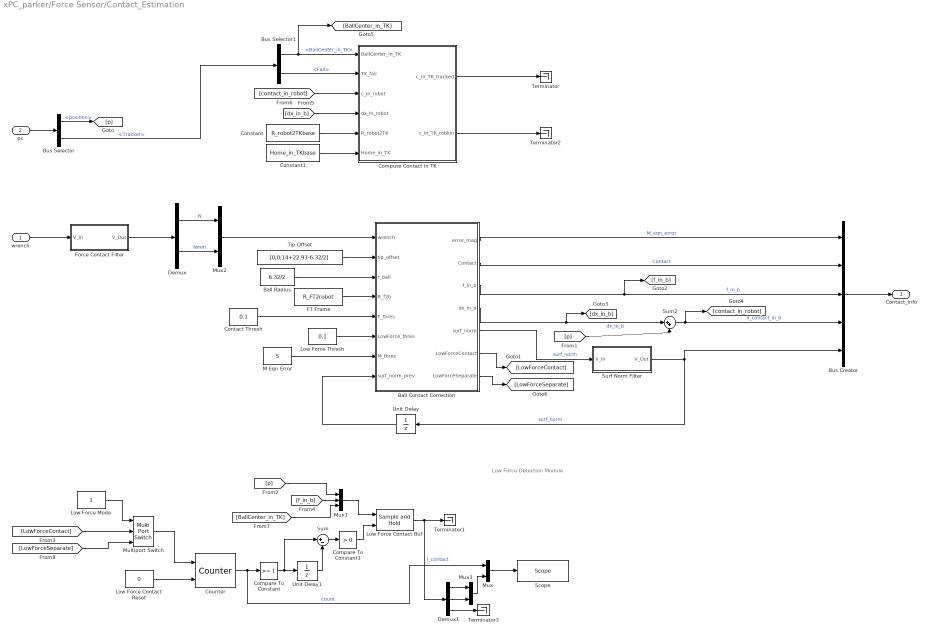
== system xPC_parker/Force Sensor/Contact_Estimation ==
  note: Low Force Detection Module
  wrench : Inport
  pc : Inport  Port=2
  Ball Contact Correction : MATLAB Function  TreatAsAtomicUnit=on
  Ball Radius : Constant  Value=6.32/2
  Bus Creator : BusCreator  Inputs=5
  Bus Selector : BusSelector  OutputSignals=position,Tracker
  Bus Selector1 : BusSelector  OutputSignals=BallCenter_in_TK,Fail
  Compare To Constant : simulink/Logic and Bit Operations/Compare To Constant  relop=>=  const=1  OutDataTypeStr=boolean
  Compare To Constant1 : simulink/Logic and Bit Operations/Compare To Constant  relop=>  const=0  OutDataTypeStr=boolean
  Compute Contact in TK : MATLAB Function  TreatAsAtomicUnit=on
  Constant : Constant  Value=R_robot2TKbase
  Constant1 : Constant  Value=Home_in_TKbase
  Contact Thresh : Constant  Value=0.1
  Counter : dspswit3/Counter  Direction=Up  CountEvent=Rising edge  CounterSize=32 bits  MaxCount=255  InitialCount=0  Output=Count  HitValue=32  ResetInput=on  SamplesPerFrame=1  Ts=1  CntDtype=double  HitDtype=Logical
  Demux : Demux  Outputs=2
  Demux1 : Demux  Outputs=[3,3,3]
  FT Frame : Constant  Value=R_FT2robot
  Force Contact Filter : Subsystem
  Low Force Contact Buf : powerlib_meascontrol/Additional Components/Sample and Hold  ic=zeros(9,1)  Ts=dt
  Low Force Contact Reset : Constant  Value=0
  Low Force Mode : Constant
  Low Force Thresh : Constant  Value=0.1
  M Eqn Error : Constant  Value=5
  Multiport Switch : MultiPortSwitch  Inputs=2
  Mux : Mux  Inputs=2
  Mux1 : Mux  Inputs=3
  Mux2 : Mux  Inputs=2
  Mux3 : Mux  Inputs=2
  "Scope " : slrtlib/Displays and Logging/Scope   scopeno=20  scopetype=Target  autostart=on  viewmode=Numerical  formatstr=Scope_format_LowForceContact  grid=on  ylimits=[0,0]  nosamples=25  noprepostsamples=0  interleave=1  triggermode=FreeRun  triggersignal=1  trigsignalfromport=off  triggerlevel=0.0  triggerslope=Either  triggerscope=1  triggersample=0  filename=data.dat  mode=Lazy  writesize=512  autorestart=off  dynamicfilemode=off  maxwritefilesize=512*1024^2
  Sum : Sum  Inputs=|+-
  Sum2 : Sum  Inputs=|++  SampleTime=dts
  Surf Norm Filter : Subsystem
  Terminator{,1..3} (4 alike) : Terminator
  Tip Offset : Constant  Value=[0;0;14+22.93-6.32/2]
  Unit Delay : UnitDelay  InitialCondition=[0;0;1]  SampleTime=-1
  Unit Delay1 : UnitDelay  SampleTime=-1
  Contact_info : Outport
  wires:
  Ball Contact Correction/2(Contact) -> Bus Creator/2  "Contact"
  FT Frame/1 -> Ball Contact Correction/4(R_f2b)
  Ball Contact Correction/1(error_mag) -> Bus Creator/1  "M_eqn_error"
  Ball Contact Correction/5(surf_norm) -> Surf Norm Filter/1(V_in)  "surf_norm"
  Ball Contact Correction/3(f_in_b) -> [f_in_b], Bus Creator/3  "f_in_b"
  Ball Radius/1 -> Ball Contact Correction/3(r_ball)
  Tip Offset/1 -> Ball Contact Correction/2(tip_offset)
  Bus Creator/1 -> Contact_info/1
  wrench/1 -> Force Contact Filter/1(V_in)
  Ball Contact Correction/4(dx_in_b) -> [dx_in_b], Sum2/1  "dx_in_b"
  Sum2/1 -> Bus Creator/4, [contact_in_robot]  "x_contact_in_b"
  Contact Thresh/1 -> Ball Contact Correction/5(F_thres)
  M Eqn Error/1 -> Ball Contact Correction/7(M_thres)
  [p] -> Sum2/2
  Force Contact Filter/1(V_Out) -> Demux/1
  Demux/2 -> Mux2/2  "Nmm"
  pc/1 -> Bus Selector/1
  Demux/1 -> Mux2/1  "N"
  Mux2/1 -> Ball Contact Correction/1(wrench)
  Bus Selector/1 -> [p]  "<position>"
  Surf Norm Filter/1(V_Out) -> Unit Delay/1, Bus Creator/5  "surf_norm"
  Unit Delay/1 -> Ball Contact Correction/8(surf_norm_prev)
  Low Force Thresh/1 -> Ball Contact Correction/6(LowForce_thres)
  Ball Contact Correction/6(LowForceContact) -> [LowForceContact]
  Low Force Contact Buf/1 -> Demux1/1, Terminator1/1  "l_contact"
  Low Force Contact Reset/1 -> Counter/2
  Mux/1 -> "Scope "/1
  Counter/1 -> Mux/1, Compare To Constant/1  "count"
  Unit Delay1/1 -> Sum/2
  Compare To Constant/1 -> Sum/1, Unit Delay1/1
  Sum/1 -> Compare To Constant1/1
  Compare To Constant1/1 -> Low Force Contact Buf/2
  [p] -> Mux1/1
  [f_in_b] -> Mux1/2
  Mux1/1 -> Low Force Contact Buf/1
  Bus Selector/2 -> Bus Selector1/1  "<Tracker>"
  Bus Selector1/1 -> [BallCenter_in_TK], Compute Contact in TK/1(BallCenter_in_TK)  "<BallCenter_in_TK>"
  Bus Selector1/2 -> Compute Contact in TK/2(TK_fail)  "<Fail>"
  [dx_in_b] -> Compute Contact in TK/4(dx_in_robot)
  Constant/1 -> Compute Contact in TK/5(R_robot2TK)
  Constant1/1 -> Compute Contact in TK/6(Home_in_TK)
  [contact_in_robot] -> Compute Contact in TK/3(c_in_robot)
  Compute Contact in TK/1(c_in_TK_tracked) -> Terminator/1
  Compute Contact in TK/2(c_in_TK_robkin) -> Terminator2/1
  [BallCenter_in_TK] -> Mux1/3
  Demux1/1 -> Mux3/1
  Demux1/2 -> Mux3/2
  Mux3/1 -> Mux/2
  Demux1/3 -> Terminator3/1
  Ball Contact Correction/7(LowForceSeparate) -> [LowForceSeparate]
  [LowForceSeparate] -> Multiport Switch/3
  [LowForceContact] -> Multiport Switch/2
  Multiport Switch/1 -> Counter/1
  Low Force Mode/1 -> Multiport Switch/1

== system xPC_parker/Force Sensor/Data_to_CMU ==
  Contact : Inport
  Bus Selector1 : BusSelector  OutputSignals=M_eqn_error,Contact,f_in_b,x_contact_in_b
  Constant : Constant  Value=UDP_EN_Data2CMU
  Mux1 : Mux  Inputs=5
  UDP : Subsystem
  tag scope: Scope_Data_to_CMU=global
  wires:
  UDP/1(delay in ms) -> Mux1/5
  Mux1/1 -> [Scope_Data_to_CMU]
  Bus Selector1/1 -> Mux1/1  "<M_eqn_error>"
  Bus Selector1/2 -> [Contact]  "<Contact>"
  [Contact] -> Mux1/2
  Bus Selector1/3 -> [f_in_b]  "<f_in_b>"
  [f_in_b] -> Mux1/3
  Bus Selector1/4 -> [x_Contact]  "<x_contact_in_b>"
  [x_Contact] -> Mux1/4
  Contact/1 -> Bus Selector1/1
  [Contact] -> UDP/1(In1)
  [f_in_b] -> UDP/2(In2)
  [x_Contact] -> UDP/3(In3)
  Constant/1 -> UDP/Enable

== system xPC_parker/Force Sensor/Dynamic Analysis ==
  wrench : Inport
  pc : Inport  Port=2
  Bus Creator : BusCreator  Inputs=5
  Bus Selector : BusSelector  OutputSignals=position
  Demux : Demux  Outputs=2
  Discrete Derivative1 : simulink/Discrete/Discrete Derivative  gainval=1.0  ICPrevScaledInput=[0;0;0]  InputProcessing=Inherited  OutMin=[]  OutMax=[]  OutDataType=fixdt(1, 16)  OutScaling=2^-10  DoSatur=off
  Discrete Derivative2 : simulink/Discrete/Discrete Derivative  gainval=1.0  ICPrevScaledInput=[0;0;0]  InputProcessing=Inherited  OutMin=[]  OutMax=[]  OutDataType=fixdt(1, 16)  OutScaling=2^-10  DoSatur=off
  Dynamic Info : Outport
  wires:
  Bus Creator/1 -> Dynamic Info/1
  wrench/1 -> Demux/1
  pc/1 -> Bus Selector/1
  Bus Selector/1 -> Bus Creator/3, Discrete Derivative1/1  "<position>"
  Demux/1 -> Bus Creator/1  "Force"
  Demux/2 -> Bus Creator/2  "Torque"
  Discrete Derivative1/1 -> Discrete Derivative2/1, Bus Creator/4  "velocity"
  Discrete Derivative2/1 -> Bus Creator/5  "acceleration"

== system xPC_parker/Force Sensor/Force Stop ==
  ResetFlag : Inport
  In1 : Inport  Port=2
  Abs : Abs
  Compare To Constant2 : simulink/Logic and Bit Operations/Compare To Constant  relop=>=  const=SafetyMargin*Wrench_max  OutDataTypeStr=boolean
  Gain : Gain
  MATLAB Function : MATLAB Function  TreatAsAtomicUnit=on
  Product : Product
  Stop Simulation : Stop
  wires:
  Abs/1 -> Gain/1
  Gain/1 -> Compare To Constant2/1
  Compare To Constant2/1 -> Stop Simulation/1
  In1/1 -> Product/1
  Product/1 -> Abs/1
  ResetFlag/1 -> MATLAB Function/1(u)
  MATLAB Function/1(y) -> Product/2

== system xPC_parker/Force Sensor/Reset Logic ==
  Reset : Inport
  Const1 : Constant
  Const2 : Constant  Value=0
  Const3 : Constant  Value=0
  N-Sample Switch : dspswit3/N-Sample Switch  N=FT_unbias_time/dts  reset=on  TriggerType=Rising edge  Ts=dts
  N-Sample Switch1 : dspswit3/N-Sample Switch  N=1  reset=off  TriggerType=Rising edge  Ts=dts
  Flag : Outport
  wires:
  Const1/1 -> N-Sample Switch/1
  N-Sample Switch/1 -> Flag/1
  Const2/1 -> N-Sample Switch/2
  Reset/1 -> N-Sample Switch1/2
  N-Sample Switch1/1 -> N-Sample Switch/3
  Const3/1 -> N-Sample Switch1/1

== system xPC_parker/Force Sensor/UDP Contact Data Log ==
  Contact : Inport
  Enable : EnablePort
  Bus Selector1 : BusSelector  OutputSignals=Contact,f_in_b,x_contact_in_b,surf_norm
  Demux1 : Demux  Outputs=12
  Digital Clock : DigitalClock  SampleTime=dtudp
  Mux3 : Mux  Inputs=6
  Pack : xpcobsoletelib/Utilities/Pack   datatypes={'double' 'double' 'double' 'double' 'double' 'double' 'double' 'double' 'double' 'double' 'double' 'double'}  byteAlign=1
  Parker_Send_to_Visual : xpcrtudplib/Legacy UDP/Send   ipAddress=255.255.255.255  ipPort=UDP_PORT_DataSend2Visual  localPort=-1  vblLen=off  sampletime=dtUDP_Data
  Rate Transition2 : RateTransition  OutPortSampleTime=dtUDP_Data
  STOP : Constant  Value=UDP_STOP
  wires:
  Pack/1 -> Parker_Send_to_Visual/1
  Mux3/1 -> Rate Transition2/1
  Rate Transition2/1 -> Demux1/1
  Demux1/1 -> Pack/1
  Demux1/2 -> Pack/2
  Demux1/3 -> Pack/3
  Demux1/4 -> Pack/4
  Demux1/5 -> Pack/5
  Demux1/6 -> Pack/6
  Demux1/7 -> Pack/7
  Demux1/8 -> Pack/8
  Bus Selector1/1 -> Mux3/1  "<Contact>"
  Bus Selector1/2 -> Mux3/2  "<f_in_b>"
  Bus Selector1/3 -> Mux3/3  "<x_contact_in_b>"
  Contact/1 -> Bus Selector1/1
  Bus Selector1/4 -> Mux3/4  "<surf_norm>"
  Demux1/9 -> Pack/9
  Demux1/10 -> Pack/10
  Digital Clock/1 -> Mux3/5
  Demux1/11 -> Pack/11
  STOP/1 -> Mux3/6
  Demux1/12 -> Pack/12

== system xPC_parker/Force Sensor/UDP Dynamic Data Log ==
  Dynamic Data : Inport
  Enable : EnablePort
  Bus Selector1 : BusSelector  OutputSignals=Force,Torque,position,velocity,acceleration
  Demux1 : Demux  Outputs=16
  Mux3 : Mux  Inputs=6
  Pack : xpcobsoletelib/Utilities/Pack   datatypes={'double' 'double' 'double' 'double' 'double' 'double' 'double' 'double' 'double' 'double' 'double' 'double' 'double' 'double' 'double' 'double'}  byteAlign=1
  Parker_Send_to_DynAna : xpcrtudplib/Legacy UDP/Send   ipAddress=255.255.255.255  ipPort=UDP_PORT_DataSend2DynAna  localPort=-1  vblLen=off  sampletime=dtUDP_Data
  Rate Transition2 : RateTransition  OutPortSampleTime=dtUDP_Data
  STOP : Constant  Value=UDP_STOP
  wires:
  Demux1/12 -> Pack/12
  STOP/1 -> Mux3/6
  Demux1/11 -> Pack/11
  Demux1/10 -> Pack/10
  Demux1/9 -> Pack/9
  Bus Selector1/4 -> Mux3/4  "<velocity>"
  Dynamic Data/1 -> Bus Selector1/1
  Bus Selector1/3 -> Mux3/3  "<position>"
  Bus Selector1/2 -> Mux3/2  "<Torque>"
  Bus Selector1/1 -> Mux3/1  "<Force>"
  Demux1/8 -> Pack/8
  Demux1/7 -> Pack/7
  Demux1/6 -> Pack/6
  Demux1/5 -> Pack/5
  Demux1/4 -> Pack/4
  Demux1/3 -> Pack/3
  Demux1/2 -> Pack/2
  Demux1/1 -> Pack/1
  Rate Transition2/1 -> Demux1/1
  Mux3/1 -> Rate Transition2/1
  Pack/1 -> Parker_Send_to_DynAna/1
  Bus Selector1/5 -> Mux3/5  "<acceleration>"
  Demux1/13 -> Pack/13
  Demux1/14 -> Pack/14
  Demux1/15 -> Pack/15
  Demux1/16 -> Pack/16

== system xPC_parker/Force Sensor/Voltage Filter Bias ==
  V_in : Inport  SampleTime=dts
  Discrete FIR Filter : DiscreteFir  CoefSource=Input port  SampleTime=dts  AccumDataTypeStr=Inherit: Same as product output
  Gain : Gain  Gain=1/N_bias  SampleTime=dts
  filter_coeffs : Constant  Value=filter_coeffs_bias  SampleTime=dts
  V_Out : Outport  SampleTime=dts
  wires:
  Gain/1 -> V_Out/1
  filter_coeffs/1 -> Discrete FIR Filter/2
  Discrete FIR Filter/1 -> Gain/1
  V_in/1 -> Discrete FIR Filter/1

== system xPC_parker/Force Sensor/Voltage Filter M AV ==
  V_in : Inport  SampleTime=dts
  Discrete FIR Filter : DiscreteFir  CoefSource=Input port  SampleTime=dts  AccumDataTypeStr=Inherit: Same as product output
  Gain : Gain  Gain=1/(dt/dts)  SampleTime=dts
  filter_coeffs : Constant  Value=ones(dt/dts,1)  SampleTime=dts
  V_Out : Outport  SampleTime=dts
  wires:
  V_in/1 -> Discrete FIR Filter/1
  Discrete FIR Filter/1 -> Gain/1
  filter_coeffs/1 -> Discrete FIR Filter/2
  Gain/1 -> V_Out/1

== system xPC_parker/Hybrid Motion PD Inverse Dynamics/Force Projector 1 ==
  Fa : Inport
  n : Inport  Port=2
  Projector : MATLAB Function  TreatAsAtomicUnit=on
  Out1 : Outport
  wires:
  Projector/1(y) -> Out1/1
  Fa/1 -> Projector/1(F)
  n/1 -> Projector/2(N)

== system xPC_parker/Hybrid Motion PD Inverse Dynamics/Force Projector 2 ==
  n : Inport
  Fa : Inport  Port=2
  Projector : MATLAB Function  TreatAsAtomicUnit=on
  Out1 : Outport
  wires:
  n/1 -> Projector/2(N)
  Fa/1 -> Projector/1(F)
  Projector/1(y) -> Out1/1

== system xPC_parker/Hybrid Motion PD Inverse Dynamics/Force Projector 3 ==
  n : Inport
  ef : Inport  Port=2
  Projector : MATLAB Function  TreatAsAtomicUnit=on
  Out1 : Outport
  wires:
  n/1 -> Projector/2(N)
  ef/1 -> Projector/1(F)
  Projector/1(y) -> Out1/1

== system xPC_parker/Hybrid Motion PD Inverse Dynamics/Motion Projector ==
  n : Inport
  Fm : Inport  Port=2
  Projector : MATLAB Function  TreatAsAtomicUnit=on
  Out1 : Outport
  wires:
  n/1 -> Projector/2(N)
  Projector/1(y) -> Out1/1
  Fm/1 -> Projector/1(F)

== system xPC_parker/Hybrid Motion PD Inverse Dynamics/Smooth Sign Function ==
  In1 : Inport
  Gain : Gain  Gain=20
  Saturation : Saturate  UpperLimit=0.05  LowerLimit=0
  Out1 : Outport
  wires:
  Saturation/1 -> Gain/1
  In1/1 -> Saturation/1
  Gain/1 -> Out1/1

== system xPC_parker/Hybrid Motion PD Inverse Dynamics/Surf Norm Command ==
  surf_norm : Inport
  Contact : Inport  Port=2
  Default_norm : Inport  Port=3
  Conflict Check : Subsystem
  Switch : Switch  Criteria=u2 > Threshold
  Out : Outport
  wires:
  Switch/1 -> Out/1
  Contact/1 -> Switch/2
  Default_norm/1 -> Conflict Check/2(default), Switch/3
  surf_norm/1 -> Conflict Check/1(surf_norm)
  Conflict Check/1(Out1) -> Switch/1

== system xPC_parker/Parker 404XR/Count to Position ==
  note: Position in mm
  count : Inport
  EncoderReset : Inport  Port=2
  Accel Filter : Subsystem
  Add : Sum  Inputs=+-
  Constant : Constant  Value=counter_offset
  Gain_Rads : Gain  Gain=2*pi/(quadrature_mode*encoder_counts)
  Position Filter observer : Subsystem
  Position Filter observer1 : Subsystem
  Rads_mm : Gain  Gain=screw_pitch/(2*pi)
  Rate Transition : RateTransition  OutPortSampleTime=dt
  Rate Transition1 : RateTransition  OutPortSampleTime=dt
  Rate Transition2 : RateTransition  OutPortSampleTime=dt
  Sample and Hold : powerlib_meascontrol/Additional Components/Sample and Hold  ic=zeros(3,1)  Ts=dt
  Subtract : Sum  Inputs=+-
  Unit Delay : UnitDelay  SampleTime=-1
  Velocity Filter : Subsystem
  Velocity Filter observer : Subsystem
  position : Outport
  velocity : Outport  Port=2
  acceleration : Outport  Port=3
  wires:
  Constant/1 -> Subtract/2
  count/1 -> Subtract/1
  Subtract/1 -> Gain_Rads/1
  Gain_Rads/1 -> Rads_mm/1
  Add/1 -> position/1
  Rads_mm/1 -> Rate Transition/1, Position Filter observer1/1(current_position), Position Filter observer/1(current_position)
  Velocity Filter/1(vel_out) -> Rate Transition1/1
  Accel Filter/1(accel_out) -> Rate Transition2/1
  Velocity Filter observer/1(vel_out) -> Accel Filter/1(velocity)
  Position Filter observer/1(vel_out) -> Velocity Filter observer/1(current_position)
  Position Filter observer1/1(vel_out) -> Velocity Filter/1(current_position)
  Sample and Hold/1 -> Unit Delay/1
  Rate Transition/1 -> Sample and Hold/1, Add/1
  Rate Transition1/1 -> velocity/1
  Rate Transition2/1 -> acceleration/1
  EncoderReset/1 -> Sample and Hold/2
  Unit Delay/1 -> Add/2

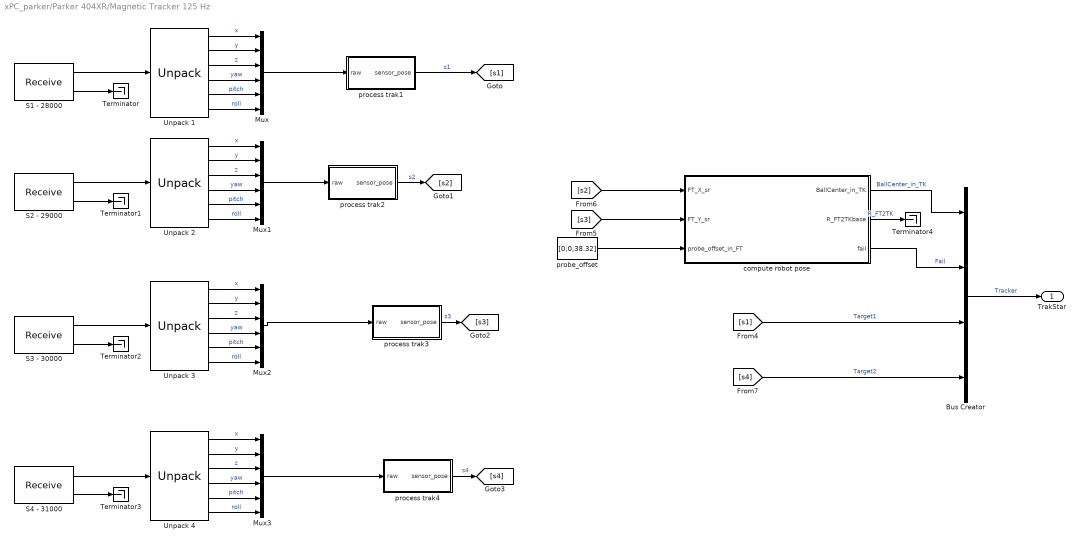
== system xPC_parker/Parker 404XR/Magnetic Tracker 125 Hz ==
  Bus Creator : BusCreator
  Mux{,1..3} (4 alike) : Mux  Inputs=6
  S1 - 28000 : xpcrtudplib/Legacy UDP/Receive   ipAddress=0.0.0.0  ipPort=28000  width=48  vblLen=on  sampletime=dt_trakstar
  S2 - 29000 : xpcrtudplib/Legacy UDP/Receive   ipAddress=0.0.0.0  ipPort=29000  width=48  vblLen=on  sampletime=dt_trakstar
  S3 - 30000 : xpcrtudplib/Legacy UDP/Receive   ipAddress=0.0.0.0  ipPort=30000  width=48  vblLen=on  sampletime=dt_trakstar
  S4 - 31000 : xpcrtudplib/Legacy UDP/Receive   ipAddress=0.0.0.0  ipPort=31000  width=48  vblLen=on  sampletime=dt_trakstar
  Terminator{,1..4} (5 alike) : Terminator
  Unpack {1..4} (4 alike) : xpcobsoletelib/Utilities/Unpack   dimensions={1,1,1,1,1,1}  datatypes={'double' 'double' 'double' 'double' 'double' 'double'}  byteAlign=1
  compute robot pose : MATLAB Function  TreatAsAtomicUnit=on
  probe_offset : Constant  Value=[0;0;38.32]
  process trak1 : Subsystem
  process trak2 : Subsystem
  process trak3 : Subsystem
  process trak4 : Subsystem
  TrakStar : Outport
  wires:
  S1 - 28000/1 -> Unpack 1/1
  S1 - 28000/2 -> Terminator/1
  Unpack 1/1 -> Mux/1  "x"
  Unpack 1/2 -> Mux/2  "y"
  Unpack 1/3 -> Mux/3  "z"
  Unpack 1/4 -> Mux/4  "yaw"
  Unpack 1/5 -> Mux/5  "pitch"
  Unpack 1/6 -> Mux/6  "roll"
  Mux/1 -> process trak1/1(raw)
  S2 - 29000/1 -> Unpack 2/1
  S2 - 29000/2 -> Terminator1/1
  Unpack 2/1 -> Mux1/1  "x"
  Unpack 2/2 -> Mux1/2  "y"
  Unpack 2/3 -> Mux1/3  "z"
  Unpack 2/4 -> Mux1/4  "yaw"
  Unpack 2/5 -> Mux1/5  "pitch"
  Unpack 2/6 -> Mux1/6  "roll"
  Mux1/1 -> process trak2/1(raw)
  Bus Creator/1 -> TrakStar/1  "Tracker"
  S3 - 30000/1 -> Unpack 3/1
  S3 - 30000/2 -> Terminator2/1
  Unpack 3/1 -> Mux2/1  "x"
  Unpack 3/2 -> Mux2/2  "y"
  Unpack 3/3 -> Mux2/3  "z"
  Unpack 3/4 -> Mux2/4  "yaw"
  Unpack 3/5 -> Mux2/5  "pitch"
  Unpack 3/6 -> Mux2/6  "roll"
  Mux2/1 -> process trak3/1(raw)
  S4 - 31000/1 -> Unpack 4/1
  S4 - 31000/2 -> Terminator3/1
  Unpack 4/1 -> Mux3/1  "x"
  Unpack 4/2 -> Mux3/2  "y"
  Unpack 4/3 -> Mux3/3  "z"
  Unpack 4/4 -> Mux3/4  "yaw"
  Unpack 4/5 -> Mux3/5  "pitch"
  Unpack 4/6 -> Mux3/6  "roll"
  Mux3/1 -> process trak4/1(raw)
  process trak1/1(sensor_pose) -> [s1]  "s1"
  process trak2/1(sensor_pose) -> [s2]  "s2"
  process trak3/1(sensor_pose) -> [s3]  "s3"
  process trak4/1(sensor_pose) -> [s4]  "s4"
  [s3] -> compute robot pose/2(FT_Y_sr)
  probe_offset/1 -> compute robot pose/3(probe_offset_in_FT)
  compute robot pose/1(BallCenter_in_TK) -> Bus Creator/1  "BallCenter_in_TK"
  compute robot pose/3(fail) -> Bus Creator/2  "Fail"
  [s4] -> Bus Creator/4  "Target2"
  compute robot pose/2(R_FT2TKbase) -> Terminator4/1  "R_FT2TK"
  [s1] -> Bus Creator/3  "Target1"
  [s2] -> compute robot pose/1(FT_X_sr)
